simulink model "hw6Q3_model"  (R2021a)
settings: Solver=VariableStepAuto  StartTime=0.0  StopTime=time_end  RelTol=1e-3
values from neighbouring files (symbols this model uses):
  K_i = K_i_list(i)    [hw6Q1.m]    (also in hw6Q2.m = K_i_list(ii); hw6Q2_tony.m = K_i_list(kk); hw6Q3.m = 0.5)
  K_p = 1    [hw6Q1.m]    (also in hw6Q2.m = K_p_list(pp); hw6Q2_tony.m = K_p_list(kk); hw6Q3.m)
  T_L = 0    [hw6Q3.m]
settings Model: Creator=kaiyu  LastModifiedBy=kaiyu

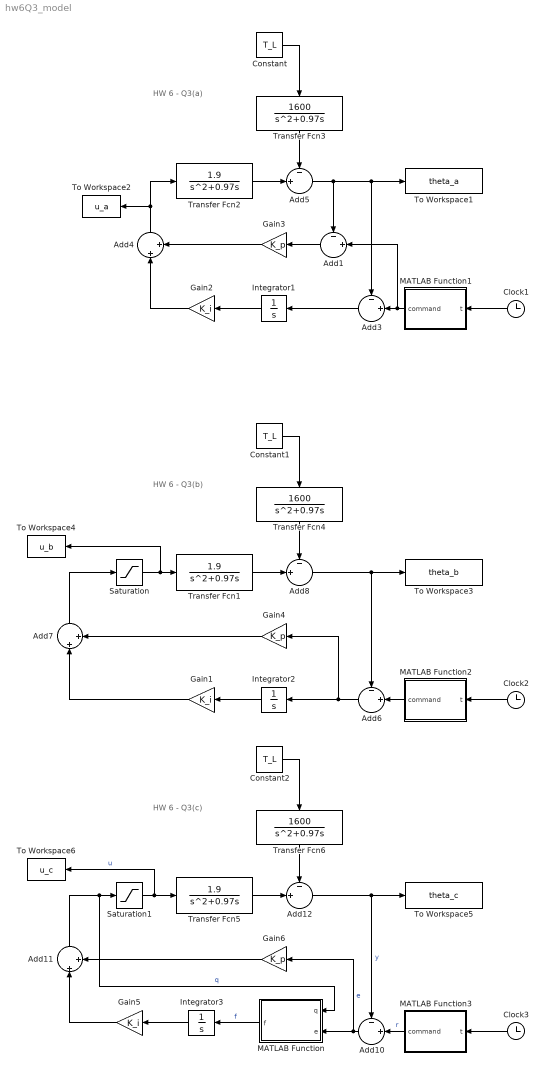
== system hw6Q3_model ==
  note: HW 6 - Q3(a)
  note: HW 6 - Q3(b)
  note: HW 6 - Q3(c)
  Add{1,3,5..6,8,10,12} (7 alike) : Sum  Inputs=-|+||
  Add11 : Sum  Inputs=||+|+
  Add4 : Sum  Inputs=||+|+
  Add7 : Sum  Inputs=||+|+
  Clock1 : Clock
  Clock2 : Clock
  Clock3 : Clock
  Constant : Constant  Value=T_L
  Constant1 : Constant  Value=T_L
  Constant2 : Constant  Value=T_L
  Gain1 : Gain  Gain=K_i
  Gain2 : Gain  Gain=K_i
  Gain3 : Gain  Gain=K_p
  Gain4 : Gain  Gain=K_p
  Gain5 : Gain  Gain=K_i
  Gain6 : Gain  Gain=K_p
  Integrator1 : Integrator
  Integrator2 : Integrator
  Integrator3 : Integrator
  MATLAB Function : MATLAB Function  TreatAsAtomicUnit=on
  MATLAB Function1 : MATLAB Function  TreatAsAtomicUnit=on
  MATLAB Function2 : MATLAB Function  TreatAsAtomicUnit=on
  MATLAB Function3 : MATLAB Function  TreatAsAtomicUnit=on
  Saturation : Saturate  UpperLimit=0.15  LowerLimit=-0.15
  Saturation1 : Saturate  UpperLimit=0.15  LowerLimit=-0.15
  To Workspace1 : ToWorkspace  VariableName=theta_a  SaveFormat=Timeseries  SampleTime=-1
  To Workspace2 : ToWorkspace  VariableName=u_a  SaveFormat=Timeseries  SampleTime=-1
  To Workspace3 : ToWorkspace  VariableName=theta_b  SaveFormat=Timeseries  SampleTime=-1
  To Workspace4 : ToWorkspace  VariableName=u_b  SaveFormat=Timeseries  SampleTime=-1
  To Workspace5 : ToWorkspace  VariableName=theta_c  SaveFormat=Timeseries  SampleTime=-1
  To Workspace6 : ToWorkspace  VariableName=u_c  SaveFormat=Timeseries  SampleTime=-1
  Transfer Fcn1 : TransferFcn  Numerator=[1.9]  Denominator=[1 0.97 0]
  Transfer Fcn2 : TransferFcn  Numerator=[1.9]  Denominator=[1 0.97 0]
  Transfer Fcn3 : TransferFcn  Numerator=[1600]  Denominator=[1 0.97 0]
  Transfer Fcn4 : TransferFcn  Numerator=[1600]  Denominator=[1 0.97 0]
  Transfer Fcn5 : TransferFcn  Numerator=[1.9]  Denominator=[1 0.97 0]
  Transfer Fcn6 : TransferFcn  Numerator=[1600]  Denominator=[1 0.97 0]
  wires:
  Add5/1 -> Add1/1, Add3/1, To Workspace1/1
  Transfer Fcn2/1 -> Add5/2
  Clock1/1 -> MATLAB Function1/1(t)
  Integrator1/1 -> Gain2/1
  Add3/1 -> Integrator1/1
  Gain3/1 -> Add4/2
  MATLAB Function1/1(command) -> Add1/2, Add3/2
  Transfer Fcn3/1 -> Add5/1
  Add4/1 -> To Workspace2/1, Transfer Fcn2/1
  Gain2/1 -> Add4/1
  Constant/1 -> Transfer Fcn3/1
  Add1/1 -> Gain3/1
  Gain1/1 -> Add7/1
  Add6/1 -> Gain4/1, Integrator2/1
  Transfer Fcn1/1 -> Add8/2
  Gain4/1 -> Add7/2
  Clock2/1 -> MATLAB Function2/1(t)
  Transfer Fcn4/1 -> Add8/1
  Add8/1 -> Add6/1, To Workspace3/1
  Constant1/1 -> Transfer Fcn4/1
  MATLAB Function2/1(command) -> Add6/2
  Integrator2/1 -> Gain1/1
  Saturation/1 -> To Workspace4/1, Transfer Fcn1/1
  Add7/1 -> Saturation/1
  Add11/1 -> MATLAB Function/1(q), Saturation1/1  "q"
  Add12/1 -> Add10/1, To Workspace5/1  "y"
  MATLAB Function3/1(command) -> Add10/2  "r"
  Constant2/1 -> Transfer Fcn6/1
  Gain6/1 -> Add11/2
  Clock3/1 -> MATLAB Function3/1(t)
  Integrator3/1 -> Gain5/1
  Transfer Fcn5/1 -> Add12/2
  Transfer Fcn6/1 -> Add12/1
  Saturation1/1 -> To Workspace6/1, Transfer Fcn5/1  "u"
  Gain5/1 -> Add11/1
  Add10/1 -> Gain6/1, MATLAB Function/2(e)  "e"
  MATLAB Function/1(f) -> Integrator3/1  "f"

== matlab function hw6Q3_model/MATLAB Function2 ==
  data: t input; command output
function command = reference(t)
if (0 <= t) && (t <= 2)
    r = 0;
else
    r = 1.0;    % radians
end
command = r;

== matlab function hw6Q3_model/MATLAB Function3 ==
  data: t input; command output
function command = reference(t)
if (0 <= t) && (t <= 2)
    r = 0;
else
    r = 1.0;    % radians
end
command = r;

== matlab function hw6Q3_model/MATLAB Function ==
  data: q input; e input; f output
function f = antiWindup(q, e)
% Actuator Saturation is at +/- 0.15 volts.
if (q >= 0.15) && (e > 0)
    output = 0;
elseif (q <= -0.15) && (e < 0)
    output = 0;
else
    output = e;
end

f = output;

== matlab function hw6Q3_model/MATLAB Function1 ==
  data: t input; command output
function command = reference(t)
if (0 <= t) && (t <= 2)
    r = 0;
else
    r = 1.0;    % radians
end
command = r;
